simulink model "UZ_EnDat_be4_diffrework"  (R2023b)
settings: Solver=FixedStepDiscrete  StartTime=0  StopTime=0.002  RelTol=1e-3
model workspace (MAT data in the model file):
  Select = 0
libraries: hdlsllib x207, simulink x17, simulink_extras x3
(part 4 of 5)

== system UZ_EnDat_be4_diffrework/UZ_ENDAT/Subsystem/stalebootupfunction ==
  CLK : Inport
  RESET : Inport  Port=2
  CLKS2DATAFLOWCHG : Inport  Port=3
  CLK2ENDOFTRANSMISSION : Inport  Port=4
  VERYSLOWCLK : Inport  Port=5
  2CLKDELAY : Delay  DelayLength=0,  DelayLengthUpperLimit=1024
  2CLKDELAY2 : Delay  DelayLength=4  DelayLengthUpperLimit=1024
  Add : Sum  OutDataTypeStr=uint32  AccumDataTypeStr=uint32
  Add1 : Sum  OutDataTypeStr=uint32  AccumDataTypeStr=uint32
  BOOTOFFSETT2 : Constant  Value=19500  OutDataTypeStr=uint32  SampleTime=-1
  BOOTOFFSETT3 : Constant  Value=97501  OutDataTypeStr=uint32  SampleTime=-1
  CLKCNTERBOOTUP : Subsystem
      settings: LibrarySourceBlock=|
      | hdlsllib/Ports &
      | Subsystems/Subsystem
  Constant : Constant  Value=0xAAAA  OutDataTypeStr=uint16  SampleTime=-1
  Constant1 : Constant  OutDataTypeStr=boolean  SampleTime=-1
  Delay : Delay  DelayLength=1
  Logical Operator : Logic  Operator=NOT  AllPortsSameDT=off  OutDataTypeStr=boolean
  Logical Operator1 : Logic  AllPortsSameDT=off  OutDataTypeStr=boolean
  Logical Operator2 : Logic  Operator=OR  Inputs=3  AllPortsSameDT=off  OutDataTypeStr=boolean
  Logical Operator3 : Logic  AllPortsSameDT=off  OutDataTypeStr=boolean
  Logical Operator4 : Logic  Operator=OR  Inputs=3  AllPortsSameDT=off  OutDataTypeStr=boolean
  Logical Operator5 : Logic  Operator=OR  AllPortsSameDT=off  OutDataTypeStr=boolean
  ManualDeserializere : Subsystem
      settings: LibrarySourceBlock=|
      | hdlsllib/Ports &
      | Subsystems/Subsystem
  OUTPUTCONTROLCONTINIOUS : Subsystem
      settings: LibrarySourceBlock=|
      | hdlsllib/Ports &
      | Subsystems/Subsystem
  Relational Operator : RelationalOperator  Operator=<=  OutDataTypeStr=boolean  InputSameDT=off
  Relational Operator1 : RelationalOperator  Operator=<=  OutDataTypeStr=boolean  InputSameDT=off
  Relational Operator2 : RelationalOperator  Operator=>  OutDataTypeStr=boolean  InputSameDT=off
  TLOWOFFSET : Constant  Value=19501  OutDataTypeStr=uint32  SampleTime=-1
  Terminator : Terminator
  CLKOUT : Outport
  DATAOUT : Outport  Port=2
  BOOTUPCOMPLETE : Outport  Port=3  OutDataTypeStr=boolean
  DATAINV : Outport  Port=4
  wires:
  CLKS2DATAFLOWCHG/1 -> Add/1
  CLK2ENDOFTRANSMISSION/1 -> Add1/1
  OUTPUTCONTROLCONTINIOUS/1(CLKOFF) -> Delay/1, Logical Operator5/1
  Logical Operator/1 -> Logical Operator1/2, OUTPUTCONTROLCONTINIOUS/4(OPENCOM)
  OUTPUTCONTROLCONTINIOUS/3(RESETCNT) -> Terminator/1
  OUTPUTCONTROLCONTINIOUS/2(DATAINV) -> DATAINV/1
  CLK/1 -> CLKCNTERBOOTUP/1(CLK), ManualDeserializere/1(CLK)
  RESET/1 -> CLKCNTERBOOTUP/3(ResetCNT), Logical Operator5/2, Logical Operator4/1
  VERYSLOWCLK/1 -> ManualDeserializere/2(SLOWCLCK), CLKCNTERBOOTUP/2(CLK2CNT), Logical Operator1/1
  Logical Operator1/1 -> Logical Operator2/1
  Delay/1 -> Logical Operator/1
  Constant/1 -> ManualDeserializere/3(DATA)
  Constant1/1 -> ManualDeserializere/5(14)
  ManualDeserializere/1(valin) -> 2CLKDELAY/1
  CLKCNTERBOOTUP/1(CNT) -> Relational Operator2/1, Relational Operator1/1, Relational Operator/1, OUTPUTCONTROLCONTINIOUS/1(CLKCNT)
  Add1/1 -> OUTPUTCONTROLCONTINIOUS/3(CLK2ENDOFTRANSMISSION)
  Add/1 -> OUTPUTCONTROLCONTINIOUS/2(CLKS2DATAFLOWCHG)
  BOOTOFFSETT2/1 -> Relational Operator/2
  Relational Operator/1 -> Logical Operator4/3, Logical Operator2/2
  Logical Operator2/1 -> CLKOUT/1
  BOOTOFFSETT3/1 -> Add/2, Add1/2, Relational Operator1/2
  TLOWOFFSET/1 -> Relational Operator2/2
  Relational Operator1/1 -> Logical Operator3/2
  Relational Operator2/1 -> Logical Operator3/1
  Logical Operator3/1 -> Logical Operator2/3, Logical Operator4/2
  Logical Operator4/1 -> ManualDeserializere/4(reset)
  Logical Operator5/1 -> 2CLKDELAY2/1
  2CLKDELAY/1 -> DATAOUT/1
  2CLKDELAY2/1 -> BOOTUPCOMPLETE/1

== system UZ_EnDat_be4_diffrework/UZ_ENDAT/Subsystem2/ManualDeserializere ==
  CLK : Inport
  SLOWCLCK : Inport  Port=2
  DATA : Inport  Port=3
  reset : Inport  Port=4
  Constant3 : Constant  Value=0  OutDataTypeStr=boolean  SampleTime=-1
  Delay1 : Delay  DelayLength=1
  Multiport Switch : MultiPortSwitch  Inputs=6  DataPortForDefault=Additional data port  DiagnosticForDefault=None  SaturateOnIntegerOverflow=off  InputSameDT=off
  Terminator{1..10} (10 alike) : Terminator
  WORDTOBOOL : Subsystem  TreatAsAtomicUnit=on
  ramwatcher : Subsystem  TreatAsAtomicUnit=on
      settings: LibrarySourceBlock=|
      | hdlsllib/Ports &
      | Subsystems/Triggered
      | Subsystem
  valin : Outport
  wires:
  SLOWCLCK/1 -> ramwatcher/Trigger
  DATA/1 -> WORDTOBOOL/1(DATAIN)
  Multiport Switch/1 -> valin/1
  CLK/1 -> WORDTOBOOL/Trigger
  Delay1/1 -> ramwatcher/1(In1)
  Constant3/1 -> Multiport Switch/8
  reset/1 -> ramwatcher/2(reset)
  WORDTOBOOL/1(DATAOUT0) -> Multiport Switch/7
  WORDTOBOOL/2(DATAOUT1) -> Multiport Switch/6
  WORDTOBOOL/3(DATAOUT2) -> Multiport Switch/5
  WORDTOBOOL/4(DATAOUT3) -> Multiport Switch/4
  WORDTOBOOL/5(DATAOUT4) -> Multiport Switch/3
  WORDTOBOOL/6(DATAOUT5) -> Multiport Switch/2
  WORDTOBOOL/9(DATAOUT8) -> Terminator2/1
  WORDTOBOOL/10(DATAOUT9) -> Terminator3/1
  WORDTOBOOL/11(DATAOUT10) -> Terminator4/1
  WORDTOBOOL/12(DATAOUT11) -> Terminator5/1
  WORDTOBOOL/13(DATAOUT12) -> Terminator6/1
  WORDTOBOOL/14(DATAOUT13) -> Terminator7/1
  WORDTOBOOL/15(DATAOUT14) -> Terminator8/1
  WORDTOBOOL/16(DATAOUT15) -> Terminator9/1
  WORDTOBOOL/7(DATAOUT6) -> Terminator1/1
  WORDTOBOOL/8(DATAOUT7) -> Terminator10/1
  ramwatcher/1(SEL) -> Multiport Switch/1, Delay1/1

== system UZ_EnDat_be4_diffrework/UZ_ENDAT/responseslicer5/ENDAT23BITREVERSER ==
  in : Inport
  32BITREVERSE : Subsystem
  Bit Shift : hdlsllib/Logic and Bit Operations/Bit Shift  mode=Shift Right Logical  N=8
  Data Type Conversion : DataTypeConversion  OutDataTypeStr=uint32  RndMeth=Nearest  SaturateOnIntegerOverflow=off
  out : Outport
  wires:
  Bit Shift/1 -> out/1
  in/1 -> Data Type Conversion/1
  32BITREVERSE/1(out) -> Bit Shift/1
  Data Type Conversion/1 -> 32BITREVERSE/1(in)

== system UZ_EnDat_be4_diffrework/UZ_ENDAT/timingprovider/CLKCNTER_POSCNTR ==
  CLK : Inport
  CLK2CNT : Inport  Port=2
  ResetCNT : Inport  Port=3  OutDataTypeStr=boolean
  Delay1 : Delay  DelayLength=1
  Positional_Counter : Subsystem  TreatAsAtomicUnit=on
      settings: LibrarySourceBlock=|
      | hdlsllib/Ports &
      | Subsystems/Triggered
      | Subsystem
  SetZero32 : Subsystem  Commented=on
  SetZero32modified : Subsystem
  SetZero32modified1 : Subsystem
  CNT : Outport
  wires:
  CLK2CNT/1 -> Positional_Counter/Trigger
  Delay1/1 -> SetZero32modified1/1(valin), CNT/1
  SetZero32modified/1(valueout) -> Delay1/1
  CLK/1 -> SetZero32modified1/Trigger, SetZero32modified/Trigger
  Positional_Counter/1(divider) -> SetZero32modified/1(valin)
  ResetCNT/1 -> SetZero32modified1/2(setzero), SetZero32modified/2(setzero)
  SetZero32modified1/1(valueout) -> Positional_Counter/1(valueout)

== system UZ_EnDat_be4_diffrework/UZ_ENDAT/timingprovider/CLKCNTER_POSCNTR1 ==
  CLK : Inport
  CLK2CNT : Inport  Port=2
  ResetCNT : Inport  Port=3  OutDataTypeStr=boolean
  Delay1 : Delay  DelayLength=1
  Positional_Counter : Subsystem  TreatAsAtomicUnit=on
      settings: LibrarySourceBlock=|
      | hdlsllib/Ports &
      | Subsystems/Triggered
      | Subsystem
  SetZero32 : Subsystem  Commented=on
  SetZero32modified : Subsystem
  CNT : Outport
  wires:
  CLK2CNT/1 -> Positional_Counter/Trigger
  SetZero32modified/1(valueout) -> Delay1/1
  CLK/1 -> SetZero32modified/Trigger
  Positional_Counter/1(divider) -> SetZero32modified/1(valin)
  ResetCNT/1 -> SetZero32modified/2(setzero)
  Delay1/1 -> Positional_Counter/1(valueout), CNT/1

== system UZ_EnDat_be4_diffrework/UZ_ENDAT/timingprovider/Subsystem ==
  elapsed : Inport
  clkcnt : Inport  Port=2
  Compare To Constant1 : hdlsllib/Logic and Bit Operations/Compare To Constant  relop===  const=5  OutDataTypeStr=boolean
  Constant : Constant  Value=20  OutDataTypeStr=uint32  SampleTime=-1
  Delay1 : Delay  DelayLength=1
  Detect Increase : simulink/Logic and Bit Operations/Detect Increase  vinit=0.0  OutDataTypeStr=boolean
      settings: LibrarySourceBlock=|
      | hdlsllib/Logic and Bit
      | Operations/Detect
      | Increase
  Switch : Switch  Criteria=u2 > Threshold  SaturateOnIntegerOverflow=off  InputSameDT=off
  nsproduct : Product  OutDataTypeStr=uint32  RndMeth=Simplest  SaturateOnIntegerOverflow=on
  ns elapsed : Outport
  wires:
  Detect Increase/1 -> Switch/2
  clkcnt/1 -> Switch/1
  Switch/1 -> nsproduct/2, Delay1/1
  Delay1/1 -> Switch/3
  elapsed/1 -> Compare To Constant1/1
  nsproduct/1 -> ns elapsed/1  "ns elapsed"
  Constant/1 -> nsproduct/1
  Compare To Constant1/1 -> Detect Increase/1

== system UZ_EnDat_be4_diffrework/UZ_ENDAT/timingprovider/Subsystem1 ==
  elapsed : Inport
  clkcnt : Inport  Port=2
  Compare To Constant1 : hdlsllib/Logic and Bit Operations/Compare To Constant  relop===  const=4  OutDataTypeStr=boolean
  Constant : Constant  Value=20  OutDataTypeStr=uint32  SampleTime=-1
  Delay1 : Delay  DelayLength=1
  Detect Increase : simulink/Logic and Bit Operations/Detect Increase  vinit=0.0  OutDataTypeStr=boolean
      settings: LibrarySourceBlock=|
      | hdlsllib/Logic and Bit
      | Operations/Detect
      | Increase
  Switch : Switch  Criteria=u2 > Threshold  SaturateOnIntegerOverflow=off  InputSameDT=off
  nsproduct : Product  OutDataTypeStr=uint32  RndMeth=Simplest  SaturateOnIntegerOverflow=on
  ns elapsed : Outport
  wires:
  Detect Increase/1 -> Switch/2
  clkcnt/1 -> Switch/1
  Switch/1 -> nsproduct/2, Delay1/1
  Delay1/1 -> Switch/3
  elapsed/1 -> Compare To Constant1/1
  nsproduct/1 -> ns elapsed/1  "ns elapsed"
  Constant/1 -> nsproduct/1
  Compare To Constant1/1 -> Detect Increase/1

== system UZ_EnDat_be4_diffrework/UZ_ENDAT/timingprovider/Subsystem2 ==
  elapsed : Inport
  clkcnt : Inport  Port=2
  Compare To Constant1 : hdlsllib/Logic and Bit Operations/Compare To Constant  relop===  const=3  OutDataTypeStr=boolean
  Constant : Constant  Value=20  OutDataTypeStr=uint32  SampleTime=-1
  Delay1 : Delay  DelayLength=1
  Detect Increase : simulink/Logic and Bit Operations/Detect Increase  vinit=0.0  OutDataTypeStr=boolean
      settings: LibrarySourceBlock=|
      | hdlsllib/Logic and Bit
      | Operations/Detect
      | Increase
  Switch : Switch  Criteria=u2 > Threshold  SaturateOnIntegerOverflow=off  InputSameDT=off
  nsproduct : Product  OutDataTypeStr=uint32  RndMeth=Simplest  SaturateOnIntegerOverflow=on
  ns elapsed : Outport
  wires:
  Detect Increase/1 -> Switch/2
  clkcnt/1 -> Switch/1
  Switch/1 -> nsproduct/2, Delay1/1
  Delay1/1 -> Switch/3
  elapsed/1 -> Compare To Constant1/1
  nsproduct/1 -> ns elapsed/1  "ns elapsed"
  Constant/1 -> nsproduct/1
  Compare To Constant1/1 -> Detect Increase/1

== system UZ_EnDat_be4_diffrework/UZ_ENDAT/timingprovider/Subsystem3 ==
  elapsed : Inport
  clkcnt : Inport  Port=2
  Compare To Constant1 : hdlsllib/Logic and Bit Operations/Compare To Constant  relop===  const=2  OutDataTypeStr=boolean
  Constant : Constant  Value=20  OutDataTypeStr=uint32  SampleTime=-1
  Delay1 : Delay  DelayLength=1
  Detect Increase : simulink/Logic and Bit Operations/Detect Increase  vinit=0.0  OutDataTypeStr=boolean
      settings: LibrarySourceBlock=|
      | hdlsllib/Logic and Bit
      | Operations/Detect
      | Increase
  Switch : Switch  Criteria=u2 > Threshold  SaturateOnIntegerOverflow=off  InputSameDT=off
  nsproduct : Product  OutDataTypeStr=uint32  RndMeth=Simplest  SaturateOnIntegerOverflow=on
  ns elapsed : Outport
  wires:
  Detect Increase/1 -> Switch/2
  clkcnt/1 -> Switch/1
  Switch/1 -> nsproduct/2, Delay1/1
  Delay1/1 -> Switch/3
  elapsed/1 -> Compare To Constant1/1
  nsproduct/1 -> ns elapsed/1  "ns elapsed"
  Constant/1 -> nsproduct/1
  Compare To Constant1/1 -> Detect Increase/1

== system UZ_EnDat_be4_diffrework/UZ_ENDAT/timingprovider/Subsystem4 ==
  countclk : Inport
  reset : Inport  Port=2
  Delay : Delay  DelayLength=1
  Detect Increase : simulink/Logic and Bit Operations/Detect Increase  vinit=0.0  OutDataTypeStr=boolean
      settings: LibrarySourceBlock=|
      | hdlsllib/Logic and Bit
      | Operations/Detect
      | Increase
  HDL Counter : hdlsllib/Sources/HDL Counter  CountType=Count limited  CountInit=0  CountStep=1  CountMax=214748364  CountFromType=Initial value  CountFrom=0  CountResetPort=on  CountLoadPort=off  CountEnbPort=on  CountDirPort=off  CountHitOutputPort=off  CountDataType=Unsigned  CountWordLen=32  CountFracLen=0  CountSampTime=1
  Scope : Scope
  valin1 : Outport  InitialOutput=0
  wires:
  countclk/1 -> Detect Increase/1
  Detect Increase/1 -> HDL Counter/2
  reset/1 -> Delay/1
  HDL Counter/1 -> valin1/1, Scope/1
  Delay/1 -> HDL Counter/1

== system UZ_EnDat_be4_diffrework/UZ_ENDAT/CRC_Check/DFF1/JKFF ==
  SET : Inport
  CLK : Inport  Port=2
  J : Inport  Port=3
  RST : Inport  Port=4
  K : Inport  Port=5
  AND : Logic  Inputs=4  IconShape=distinctive  AllPortsSameDT=off  OutDataTypeStr=boolean
  AND1 : Logic  Inputs=4  IconShape=distinctive  AllPortsSameDT=off  OutDataTypeStr=boolean
  AND{2..5} (4 alike) : Logic  IconShape=distinctive  AllPortsSameDT=off  OutDataTypeStr=boolean
  Delay{,1..3} (4 alike) : Delay  DelayLength=1
  NOR : Logic  Operator=NOR  Inputs=4  IconShape=distinctive  AllPortsSameDT=off  OutDataTypeStr=boolean
  NOR1 : Logic  Operator=NOR  Inputs=4  IconShape=distinctive  AllPortsSameDT=off  OutDataTypeStr=boolean
  NOR2 : Logic  Operator=NOR  IconShape=distinctive  AllPortsSameDT=off  OutDataTypeStr=boolean
  NOR3 : Logic  Operator=NAND  IconShape=distinctive  AllPortsSameDT=off  OutDataTypeStr=boolean
  NOR4 : Logic  Operator=NOR  IconShape=distinctive  AllPortsSameDT=off  OutDataTypeStr=boolean
  NOR5 : Logic  Operator=NAND  IconShape=distinctive  AllPortsSameDT=off  OutDataTypeStr=boolean
  NOT : Logic  Operator=NOT  IconShape=distinctive  AllPortsSameDT=off  OutDataTypeStr=boolean
  NOT1 : Logic  Operator=NOT  IconShape=distinctive  AllPortsSameDT=off  OutDataTypeStr=boolean
  OR : Logic  Operator=OR  Inputs=3  IconShape=distinctive  AllPortsSameDT=off  OutDataTypeStr=boolean
  OQ : Outport
  NOQ : Outport  Port=2
  wires:
  RST/1 -> NOR4/2, NOR1/4
  J/1 -> OR/1, AND/2
  CLK/1 -> AND5/1, AND4/2, OR/2, NOT/1
  NOT/1 -> AND/3, AND1/2
  K/1 -> OR/3, AND1/3
  OR/1 -> AND1/1, NOT1/1, AND/4
  NOT1/1 -> AND2/1, AND3/2
  AND3/1 -> NOR/3
  AND/1 -> NOR/2
  AND2/1 -> NOR1/2
  AND1/1 -> NOR1/3
  SET/1 -> NOR2/1, NOR/1
  NOR/1 -> Delay/1
  NOR1/1 -> Delay1/1
  AND5/1 -> NOR2/2
  NOR2/1 -> NOR3/1
  AND4/1 -> NOR4/1
  NOR4/1 -> NOR5/2
  NOR3/1 -> Delay3/1
  NOR5/1 -> Delay2/1
  Delay/1 -> NOR1/1, AND4/1
  Delay1/1 -> NOR/4, AND5/2
  Delay2/1 -> NOR3/2, AND2/2, AND/1, NOQ/1
  Delay3/1 -> AND3/1, AND1/4, NOR5/1, OQ/1

== system UZ_EnDat_be4_diffrework/UZ_ENDAT/CRC_Check/DFF2/JKFF ==
  SET : Inport
  CLK : Inport  Port=2
  J : Inport  Port=3
  RST : Inport  Port=4
  K : Inport  Port=5
  AND : Logic  Inputs=4  IconShape=distinctive  AllPortsSameDT=off  OutDataTypeStr=boolean
  AND1 : Logic  Inputs=4  IconShape=distinctive  AllPortsSameDT=off  OutDataTypeStr=boolean
  AND{2..5} (4 alike) : Logic  IconShape=distinctive  AllPortsSameDT=off  OutDataTypeStr=boolean
  Delay{,1..3} (4 alike) : Delay  DelayLength=1
  NOR : Logic  Operator=NOR  Inputs=4  IconShape=distinctive  AllPortsSameDT=off  OutDataTypeStr=boolean
  NOR1 : Logic  Operator=NOR  Inputs=4  IconShape=distinctive  AllPortsSameDT=off  OutDataTypeStr=boolean
  NOR2 : Logic  Operator=NOR  IconShape=distinctive  AllPortsSameDT=off  OutDataTypeStr=boolean
  NOR3 : Logic  Operator=NAND  IconShape=distinctive  AllPortsSameDT=off  OutDataTypeStr=boolean
  NOR4 : Logic  Operator=NOR  IconShape=distinctive  AllPortsSameDT=off  OutDataTypeStr=boolean
  NOR5 : Logic  Operator=NAND  IconShape=distinctive  AllPortsSameDT=off  OutDataTypeStr=boolean
  NOT : Logic  Operator=NOT  IconShape=distinctive  AllPortsSameDT=off  OutDataTypeStr=boolean
  NOT1 : Logic  Operator=NOT  IconShape=distinctive  AllPortsSameDT=off  OutDataTypeStr=boolean
  OR : Logic  Operator=OR  Inputs=3  IconShape=distinctive  AllPortsSameDT=off  OutDataTypeStr=boolean
  OQ : Outport
  NOQ : Outport  Port=2
  wires:
  RST/1 -> NOR4/2, NOR1/4
  J/1 -> OR/1, AND/2
  CLK/1 -> AND5/1, AND4/2, OR/2, NOT/1
  NOT/1 -> AND/3, AND1/2
  K/1 -> OR/3, AND1/3
  OR/1 -> AND1/1, NOT1/1, AND/4
  NOT1/1 -> AND2/1, AND3/2
  AND3/1 -> NOR/3
  AND/1 -> NOR/2
  AND2/1 -> NOR1/2
  AND1/1 -> NOR1/3
  SET/1 -> NOR2/1, NOR/1
  NOR/1 -> Delay/1
  NOR1/1 -> Delay1/1
  AND5/1 -> NOR2/2
  NOR2/1 -> NOR3/1
  AND4/1 -> NOR4/1
  NOR4/1 -> NOR5/2
  NOR3/1 -> Delay3/1
  NOR5/1 -> Delay2/1
  Delay/1 -> NOR1/1, AND4/1
  Delay1/1 -> NOR/4, AND5/2
  Delay2/1 -> NOR3/2, AND2/2, AND/1, NOQ/1
  Delay3/1 -> AND3/1, AND1/4, NOR5/1, OQ/1

== system UZ_EnDat_be4_diffrework/UZ_ENDAT/CRC_Check/DFF3/JKFF ==
  SET : Inport
  CLK : Inport  Port=2
  J : Inport  Port=3
  RST : Inport  Port=4
  K : Inport  Port=5
  AND : Logic  Inputs=4  IconShape=distinctive  AllPortsSameDT=off  OutDataTypeStr=boolean
  AND1 : Logic  Inputs=4  IconShape=distinctive  AllPortsSameDT=off  OutDataTypeStr=boolean
  AND{2..5} (4 alike) : Logic  IconShape=distinctive  AllPortsSameDT=off  OutDataTypeStr=boolean
  Delay{,1..3} (4 alike) : Delay  DelayLength=1
  NOR : Logic  Operator=NOR  Inputs=4  IconShape=distinctive  AllPortsSameDT=off  OutDataTypeStr=boolean
  NOR1 : Logic  Operator=NOR  Inputs=4  IconShape=distinctive  AllPortsSameDT=off  OutDataTypeStr=boolean
  NOR2 : Logic  Operator=NOR  IconShape=distinctive  AllPortsSameDT=off  OutDataTypeStr=boolean
  NOR3 : Logic  Operator=NAND  IconShape=distinctive  AllPortsSameDT=off  OutDataTypeStr=boolean
  NOR4 : Logic  Operator=NOR  IconShape=distinctive  AllPortsSameDT=off  OutDataTypeStr=boolean
  NOR5 : Logic  Operator=NAND  IconShape=distinctive  AllPortsSameDT=off  OutDataTypeStr=boolean
  NOT : Logic  Operator=NOT  IconShape=distinctive  AllPortsSameDT=off  OutDataTypeStr=boolean
  NOT1 : Logic  Operator=NOT  IconShape=distinctive  AllPortsSameDT=off  OutDataTypeStr=boolean
  OR : Logic  Operator=OR  Inputs=3  IconShape=distinctive  AllPortsSameDT=off  OutDataTypeStr=boolean
  OQ : Outport
  NOQ : Outport  Port=2
  wires:
  RST/1 -> NOR4/2, NOR1/4
  J/1 -> OR/1, AND/2
  CLK/1 -> AND5/1, AND4/2, OR/2, NOT/1
  NOT/1 -> AND/3, AND1/2
  K/1 -> OR/3, AND1/3
  OR/1 -> AND1/1, NOT1/1, AND/4
  NOT1/1 -> AND2/1, AND3/2
  AND3/1 -> NOR/3
  AND/1 -> NOR/2
  AND2/1 -> NOR1/2
  AND1/1 -> NOR1/3
  SET/1 -> NOR2/1, NOR/1
  NOR/1 -> Delay/1
  NOR1/1 -> Delay1/1
  AND5/1 -> NOR2/2
  NOR2/1 -> NOR3/1
  AND4/1 -> NOR4/1
  NOR4/1 -> NOR5/2
  NOR3/1 -> Delay3/1
  NOR5/1 -> Delay2/1
  Delay/1 -> NOR1/1, AND4/1
  Delay1/1 -> NOR/4, AND5/2
  Delay2/1 -> NOR3/2, AND2/2, AND/1, NOQ/1
  Delay3/1 -> AND3/1, AND1/4, NOR5/1, OQ/1

== system UZ_EnDat_be4_diffrework/UZ_ENDAT/CRC_Check/DFF4/JKFF ==
  SET : Inport
  CLK : Inport  Port=2
  J : Inport  Port=3
  RST : Inport  Port=4
  K : Inport  Port=5
  AND : Logic  Inputs=4  IconShape=distinctive  AllPortsSameDT=off  OutDataTypeStr=boolean
  AND1 : Logic  Inputs=4  IconShape=distinctive  AllPortsSameDT=off  OutDataTypeStr=boolean
  AND{2..5} (4 alike) : Logic  IconShape=distinctive  AllPortsSameDT=off  OutDataTypeStr=boolean
  Delay{,1..3} (4 alike) : Delay  DelayLength=1
  NOR : Logic  Operator=NOR  Inputs=4  IconShape=distinctive  AllPortsSameDT=off  OutDataTypeStr=boolean
  NOR1 : Logic  Operator=NOR  Inputs=4  IconShape=distinctive  AllPortsSameDT=off  OutDataTypeStr=boolean
  NOR2 : Logic  Operator=NOR  IconShape=distinctive  AllPortsSameDT=off  OutDataTypeStr=boolean
  NOR3 : Logic  Operator=NAND  IconShape=distinctive  AllPortsSameDT=off  OutDataTypeStr=boolean
  NOR4 : Logic  Operator=NOR  IconShape=distinctive  AllPortsSameDT=off  OutDataTypeStr=boolean
  NOR5 : Logic  Operator=NAND  IconShape=distinctive  AllPortsSameDT=off  OutDataTypeStr=boolean
  NOT : Logic  Operator=NOT  IconShape=distinctive  AllPortsSameDT=off  OutDataTypeStr=boolean
  NOT1 : Logic  Operator=NOT  IconShape=distinctive  AllPortsSameDT=off  OutDataTypeStr=boolean
  OR : Logic  Operator=OR  Inputs=3  IconShape=distinctive  AllPortsSameDT=off  OutDataTypeStr=boolean
  OQ : Outport
  NOQ : Outport  Port=2
  wires:
  RST/1 -> NOR4/2, NOR1/4
  J/1 -> OR/1, AND/2
  CLK/1 -> AND5/1, AND4/2, OR/2, NOT/1
  NOT/1 -> AND/3, AND1/2
  K/1 -> OR/3, AND1/3
  OR/1 -> AND1/1, NOT1/1, AND/4
  NOT1/1 -> AND2/1, AND3/2
  AND3/1 -> NOR/3
  AND/1 -> NOR/2
  AND2/1 -> NOR1/2
  AND1/1 -> NOR1/3
  SET/1 -> NOR2/1, NOR/1
  NOR/1 -> Delay/1
  NOR1/1 -> Delay1/1
  AND5/1 -> NOR2/2
  NOR2/1 -> NOR3/1
  AND4/1 -> NOR4/1
  NOR4/1 -> NOR5/2
  NOR3/1 -> Delay3/1
  NOR5/1 -> Delay2/1
  Delay/1 -> NOR1/1, AND4/1
  Delay1/1 -> NOR/4, AND5/2
  Delay2/1 -> NOR3/2, AND2/2, AND/1, NOQ/1
  Delay3/1 -> AND3/1, AND1/4, NOR5/1, OQ/1

== system UZ_EnDat_be4_diffrework/UZ_ENDAT/CRC_Check/DFF5/JKFF ==
  SET : Inport
  CLK : Inport  Port=2
  J : Inport  Port=3
  RST : Inport  Port=4
  K : Inport  Port=5
  AND : Logic  Inputs=4  IconShape=distinctive  AllPortsSameDT=off  OutDataTypeStr=boolean
  AND1 : Logic  Inputs=4  IconShape=distinctive  AllPortsSameDT=off  OutDataTypeStr=boolean
  AND{2..5} (4 alike) : Logic  IconShape=distinctive  AllPortsSameDT=off  OutDataTypeStr=boolean
  Delay{,1..3} (4 alike) : Delay  DelayLength=1
  NOR : Logic  Operator=NOR  Inputs=4  IconShape=distinctive  AllPortsSameDT=off  OutDataTypeStr=boolean
  NOR1 : Logic  Operator=NOR  Inputs=4  IconShape=distinctive  AllPortsSameDT=off  OutDataTypeStr=boolean
  NOR2 : Logic  Operator=NOR  IconShape=distinctive  AllPortsSameDT=off  OutDataTypeStr=boolean
  NOR3 : Logic  Operator=NAND  IconShape=distinctive  AllPortsSameDT=off  OutDataTypeStr=boolean
  NOR4 : Logic  Operator=NOR  IconShape=distinctive  AllPortsSameDT=off  OutDataTypeStr=boolean
  NOR5 : Logic  Operator=NAND  IconShape=distinctive  AllPortsSameDT=off  OutDataTypeStr=boolean
  NOT : Logic  Operator=NOT  IconShape=distinctive  AllPortsSameDT=off  OutDataTypeStr=boolean
  NOT1 : Logic  Operator=NOT  IconShape=distinctive  AllPortsSameDT=off  OutDataTypeStr=boolean
  OR : Logic  Operator=OR  Inputs=3  IconShape=distinctive  AllPortsSameDT=off  OutDataTypeStr=boolean
  OQ : Outport
  NOQ : Outport  Port=2
  wires:
  RST/1 -> NOR4/2, NOR1/4
  J/1 -> OR/1, AND/2
  CLK/1 -> AND5/1, AND4/2, OR/2, NOT/1
  NOT/1 -> AND/3, AND1/2
  K/1 -> OR/3, AND1/3
  OR/1 -> AND1/1, NOT1/1, AND/4
  NOT1/1 -> AND2/1, AND3/2
  AND3/1 -> NOR/3
  AND/1 -> NOR/2
  AND2/1 -> NOR1/2
  AND1/1 -> NOR1/3
  SET/1 -> NOR2/1, NOR/1
  NOR/1 -> Delay/1
  NOR1/1 -> Delay1/1
  AND5/1 -> NOR2/2
  NOR2/1 -> NOR3/1
  AND4/1 -> NOR4/1
  NOR4/1 -> NOR5/2
  NOR3/1 -> Delay3/1
  NOR5/1 -> Delay2/1
  Delay/1 -> NOR1/1, AND4/1
  Delay1/1 -> NOR/4, AND5/2
  Delay2/1 -> NOR3/2, AND2/2, AND/1, NOQ/1
  Delay3/1 -> AND3/1, AND1/4, NOR5/1, OQ/1

== system UZ_EnDat_be4_diffrework/UZ_ENDAT/CRC_Check/DFF6/JKFF ==
  SET : Inport
  CLK : Inport  Port=2
  J : Inport  Port=3
  RST : Inport  Port=4
  K : Inport  Port=5
  AND : Logic  Inputs=4  IconShape=distinctive  AllPortsSameDT=off  OutDataTypeStr=boolean
  AND1 : Logic  Inputs=4  IconShape=distinctive  AllPortsSameDT=off  OutDataTypeStr=boolean
  AND{2..5} (4 alike) : Logic  IconShape=distinctive  AllPortsSameDT=off  OutDataTypeStr=boolean
  Delay{,1..3} (4 alike) : Delay  DelayLength=1
  NOR : Logic  Operator=NOR  Inputs=4  IconShape=distinctive  AllPortsSameDT=off  OutDataTypeStr=boolean
  NOR1 : Logic  Operator=NOR  Inputs=4  IconShape=distinctive  AllPortsSameDT=off  OutDataTypeStr=boolean
  NOR2 : Logic  Operator=NOR  IconShape=distinctive  AllPortsSameDT=off  OutDataTypeStr=boolean
  NOR3 : Logic  Operator=NAND  IconShape=distinctive  AllPortsSameDT=off  OutDataTypeStr=boolean
  NOR4 : Logic  Operator=NOR  IconShape=distinctive  AllPortsSameDT=off  OutDataTypeStr=boolean
  NOR5 : Logic  Operator=NAND  IconShape=distinctive  AllPortsSameDT=off  OutDataTypeStr=boolean
  NOT : Logic  Operator=NOT  IconShape=distinctive  AllPortsSameDT=off  OutDataTypeStr=boolean
  NOT1 : Logic  Operator=NOT  IconShape=distinctive  AllPortsSameDT=off  OutDataTypeStr=boolean
  OR : Logic  Operator=OR  Inputs=3  IconShape=distinctive  AllPortsSameDT=off  OutDataTypeStr=boolean
  OQ : Outport
  NOQ : Outport  Port=2
  wires:
  RST/1 -> NOR4/2, NOR1/4
  J/1 -> OR/1, AND/2
  CLK/1 -> AND5/1, AND4/2, OR/2, NOT/1
  NOT/1 -> AND/3, AND1/2
  K/1 -> OR/3, AND1/3
  OR/1 -> AND1/1, NOT1/1, AND/4
  NOT1/1 -> AND2/1, AND3/2
  AND3/1 -> NOR/3
  AND/1 -> NOR/2
  AND2/1 -> NOR1/2
  AND1/1 -> NOR1/3
  SET/1 -> NOR2/1, NOR/1
  NOR/1 -> Delay/1
  NOR1/1 -> Delay1/1
  AND5/1 -> NOR2/2
  NOR2/1 -> NOR3/1
  AND4/1 -> NOR4/1
  NOR4/1 -> NOR5/2
  NOR3/1 -> Delay3/1
  NOR5/1 -> Delay2/1
  Delay/1 -> NOR1/1, AND4/1
  Delay1/1 -> NOR/4, AND5/2
  Delay2/1 -> NOR3/2, AND2/2, AND/1, NOQ/1
  Delay3/1 -> AND3/1, AND1/4, NOR5/1, OQ/1

== system UZ_EnDat_be4_diffrework/UZ_ENDAT/INITIALOFF/CLKCNTER_FAST/Positional_Counter ==
  valueout : Inport  OutDataTypeStr=uint32
  Trigger : TriggerPort  TriggerType=either  VariantControl=(inherit)  InitialTriggerSignalState=zero
  Add : Sum  OutDataTypeStr=uint32  AccumDataTypeStr=uint32  InputSameDT=on  RndMeth=Simplest  SaturateOnIntegerOverflow=on
  Constant : Constant  OutDataTypeStr=uint32  SampleTime=-1
  divider : Outport  InitialOutput=0
  wires:
  valueout/1 -> Add/1
  Add/1 -> divider/1
  Constant/1 -> Add/2

== system UZ_EnDat_be4_diffrework/UZ_ENDAT/ManualSerialize/Storage1/prolonger ==
  in : Inport
  Delay4 : Delay  DelayLength=1
  Logical Operator5 : Logic  Operator=OR  AllPortsSameDT=off  OutDataTypeStr=boolean
  out : Outport
  wires:
  Logical Operator5/1 -> out/1
  in/1 -> Delay4/1, Logical Operator5/1
  Delay4/1 -> Logical Operator5/2

== system UZ_EnDat_be4_diffrework/UZ_ENDAT/ManualSerialize/Storage2/prolonger ==
  in : Inport
  Delay4 : Delay  DelayLength=1
  Logical Operator5 : Logic  Operator=OR  Inputs=3  AllPortsSameDT=off  OutDataTypeStr=boolean
  out : Outport
  wires:
  Logical Operator5/1 -> out/1
  in/1 -> Logical Operator5/3, Delay4/1, Logical Operator5/1
  Delay4/1 -> Logical Operator5/2

== system UZ_EnDat_be4_diffrework/UZ_ENDAT/ManualSerialize/nibblepadding6/padding ==
  in : Inport
  Bit Shift2 : hdlsllib/Logic and Bit Operations/Bit Shift  mode=Shift Right Logical  N=1
  Bit Slice2 : hdlsllib/Logic and Bit Operations/Bit Slice  lidx=0  ridx=0
  Data Type Conversion2 : DataTypeConversion  OutDataTypeStr=boolean  RndMeth=Nearest  SaturateOnIntegerOverflow=off
  Switch2 : Switch  Criteria=u2 > Threshold  SaturateOnIntegerOverflow=off  InputSameDT=off
  out : Outport
  wires:
  in/1 -> Bit Shift2/1, Switch2/1, Bit Slice2/1
  Bit Shift2/1 -> Switch2/3
  Data Type Conversion2/1 -> Switch2/2
  Bit Slice2/1 -> Data Type Conversion2/1
  Switch2/1 -> out/1

== system UZ_EnDat_be4_diffrework/UZ_ENDAT/ManualSerialize/nibblepadding6/padding1 ==
  in : Inport
  Bit Shift2 : hdlsllib/Logic and Bit Operations/Bit Shift  mode=Shift Right Logical  N=1
  Bit Slice2 : hdlsllib/Logic and Bit Operations/Bit Slice  lidx=0  ridx=0
  Data Type Conversion2 : DataTypeConversion  OutDataTypeStr=boolean  RndMeth=Nearest  SaturateOnIntegerOverflow=off
  Switch2 : Switch  Criteria=u2 > Threshold  SaturateOnIntegerOverflow=off  InputSameDT=off
  out : Outport
  wires:
  in/1 -> Bit Shift2/1, Switch2/1, Bit Slice2/1
  Bit Shift2/1 -> Switch2/3
  Data Type Conversion2/1 -> Switch2/2
  Bit Slice2/1 -> Data Type Conversion2/1
  Switch2/1 -> out/1

== system UZ_EnDat_be4_diffrework/UZ_ENDAT/ManualSerialize/nibblepadding6/padding2 ==
  in : Inport
  Bit Shift2 : hdlsllib/Logic and Bit Operations/Bit Shift  mode=Shift Right Logical  N=1
  Bit Slice2 : hdlsllib/Logic and Bit Operations/Bit Slice  lidx=0  ridx=0
  Data Type Conversion2 : DataTypeConversion  OutDataTypeStr=boolean  RndMeth=Nearest  SaturateOnIntegerOverflow=off
  Switch2 : Switch  Criteria=u2 > Threshold  SaturateOnIntegerOverflow=off  InputSameDT=off
  out : Outport
  wires:
  in/1 -> Bit Shift2/1, Switch2/1, Bit Slice2/1
  Bit Shift2/1 -> Switch2/3
  Data Type Conversion2/1 -> Switch2/2
  Bit Slice2/1 -> Data Type Conversion2/1
  Switch2/1 -> out/1

== system UZ_EnDat_be4_diffrework/UZ_ENDAT/ManualSerialize/nibblepadding6/padding3 ==
  in : Inport
  Bit Shift2 : hdlsllib/Logic and Bit Operations/Bit Shift  mode=Shift Right Logical  N=1
  Bit Slice2 : hdlsllib/Logic and Bit Operations/Bit Slice  lidx=0  ridx=0
  Data Type Conversion2 : DataTypeConversion  OutDataTypeStr=boolean  RndMeth=Nearest  SaturateOnIntegerOverflow=off
  Switch2 : Switch  Criteria=u2 > Threshold  SaturateOnIntegerOverflow=off  InputSameDT=off
  out : Outport
  wires:
  in/1 -> Bit Shift2/1, Switch2/1, Bit Slice2/1
  Bit Shift2/1 -> Switch2/3
  Data Type Conversion2/1 -> Switch2/2
  Bit Slice2/1 -> Data Type Conversion2/1
  Switch2/1 -> out/1

== system UZ_EnDat_be4_diffrework/UZ_ENDAT/RESPONSESLICER5X/19BITSLICER/responseslicer ==
  DATA : Inport  OutDataTypeStr=uint64
  Bit Slice1 : hdlsllib/Logic and Bit Operations/Bit Slice  lidx=2  ridx=2
  Bit Slice3 : hdlsllib/Logic and Bit Operations/Bit Slice  lidx=25  ridx=21
  Bit Slice4 : hdlsllib/Logic and Bit Operations/Bit Slice  lidx=20  ridx=2
  Data Type Conversion1 : DataTypeConversion  OutDataTypeStr=boolean  SaturateOnIntegerOverflow=off  RndMeth=Floor
  Data Type Conversion3 : DataTypeConversion  OutDataTypeStr=uint8  SaturateOnIntegerOverflow=off  RndMeth=Floor
  Data Type Conversion4 : DataTypeConversion  OutDataTypeStr=uint32  SaturateOnIntegerOverflow=off  RndMeth=Floor
  Terminator : Terminator
  CRC : Outport  OutDataTypeStr=uint8
  payload : Outport  Port=2  OutDataTypeStr=uint32
  error : Outport  Port=3  OutDataTypeStr=boolean
  wires:
  DATA/1 -> Terminator/1, Bit Slice1/1, Bit Slice4/1, Bit Slice3/1
  Bit Slice3/1 -> Data Type Conversion3/1
  Bit Slice4/1 -> Data Type Conversion4/1
  Data Type Conversion3/1 -> CRC/1
  Data Type Conversion4/1 -> payload/1
  Bit Slice1/1 -> Data Type Conversion1/1
  Data Type Conversion1/1 -> error/1

== system UZ_EnDat_be4_diffrework/UZ_ENDAT/RESPONSESLICER5X/19BITSLICER/responseslicer1 ==
  DATA : Inport  OutDataTypeStr=uint64
  Bit Slice1 : hdlsllib/Logic and Bit Operations/Bit Slice  lidx=2  ridx=2
  Bit Slice3 : hdlsllib/Logic and Bit Operations/Bit Slice  lidx=25  ridx=21
  Bit Slice4 : hdlsllib/Logic and Bit Operations/Bit Slice  lidx=20  ridx=2
  Data Type Conversion1 : DataTypeConversion  OutDataTypeStr=boolean  SaturateOnIntegerOverflow=off  RndMeth=Floor
  Data Type Conversion3 : DataTypeConversion  OutDataTypeStr=uint8  SaturateOnIntegerOverflow=off  RndMeth=Floor
  Data Type Conversion4 : DataTypeConversion  OutDataTypeStr=uint32  SaturateOnIntegerOverflow=off  RndMeth=Floor
  Terminator : Terminator
  CRC : Outport  OutDataTypeStr=uint8
  payload : Outport  Port=2  OutDataTypeStr=uint32
  error : Outport  Port=3  OutDataTypeStr=boolean
  wires:
  DATA/1 -> Terminator/1, Bit Slice1/1, Bit Slice4/1, Bit Slice3/1
  Bit Slice3/1 -> Data Type Conversion3/1
  Bit Slice4/1 -> Data Type Conversion4/1
  Data Type Conversion3/1 -> CRC/1
  Data Type Conversion4/1 -> payload/1
  Bit Slice1/1 -> Data Type Conversion1/1
  Data Type Conversion1/1 -> error/1

== system UZ_EnDat_be4_diffrework/UZ_ENDAT/RESPONSESLICER5X/19BITSLICER/responseslicer2 ==
  DATA : Inport  OutDataTypeStr=uint64
  Bit Slice1 : hdlsllib/Logic and Bit Operations/Bit Slice  lidx=2  ridx=2
  Bit Slice3 : hdlsllib/Logic and Bit Operations/Bit Slice  lidx=25  ridx=21
  Bit Slice4 : hdlsllib/Logic and Bit Operations/Bit Slice  lidx=20  ridx=2
  Data Type Conversion1 : DataTypeConversion  OutDataTypeStr=boolean  SaturateOnIntegerOverflow=off  RndMeth=Floor
  Data Type Conversion3 : DataTypeConversion  OutDataTypeStr=uint8  SaturateOnIntegerOverflow=off  RndMeth=Floor
  Data Type Conversion4 : DataTypeConversion  OutDataTypeStr=uint32  SaturateOnIntegerOverflow=off  RndMeth=Floor
  Terminator : Terminator
  CRC : Outport  OutDataTypeStr=uint8
  payload : Outport  Port=2  OutDataTypeStr=uint32
  error : Outport  Port=3  OutDataTypeStr=boolean
  wires:
  DATA/1 -> Terminator/1, Bit Slice1/1, Bit Slice4/1, Bit Slice3/1
  Bit Slice3/1 -> Data Type Conversion3/1
  Bit Slice4/1 -> Data Type Conversion4/1
  Data Type Conversion3/1 -> CRC/1
  Data Type Conversion4/1 -> payload/1
  Bit Slice1/1 -> Data Type Conversion1/1
  Data Type Conversion1/1 -> error/1

== system UZ_EnDat_be4_diffrework/UZ_ENDAT/RESPONSESLICER5X/19BITSLICER/responseslicer3 ==
  DATA : Inport  OutDataTypeStr=uint64
  Bit Slice1 : hdlsllib/Logic and Bit Operations/Bit Slice  lidx=2  ridx=2
  Bit Slice3 : hdlsllib/Logic and Bit Operations/Bit Slice  lidx=25  ridx=21
  Bit Slice4 : hdlsllib/Logic and Bit Operations/Bit Slice  lidx=20  ridx=2
  Data Type Conversion1 : DataTypeConversion  OutDataTypeStr=boolean  SaturateOnIntegerOverflow=off  RndMeth=Floor
  Data Type Conversion3 : DataTypeConversion  OutDataTypeStr=uint8  SaturateOnIntegerOverflow=off  RndMeth=Floor
  Data Type Conversion4 : DataTypeConversion  OutDataTypeStr=uint32  SaturateOnIntegerOverflow=off  RndMeth=Floor
  Terminator : Terminator
  CRC : Outport  OutDataTypeStr=uint8
  payload : Outport  Port=2  OutDataTypeStr=uint32
  error : Outport  Port=3  OutDataTypeStr=boolean
  wires:
  DATA/1 -> Terminator/1, Bit Slice1/1, Bit Slice4/1, Bit Slice3/1
  Bit Slice3/1 -> Data Type Conversion3/1
  Bit Slice4/1 -> Data Type Conversion4/1
  Data Type Conversion3/1 -> CRC/1
  Data Type Conversion4/1 -> payload/1
  Bit Slice1/1 -> Data Type Conversion1/1
  Data Type Conversion1/1 -> error/1

== system UZ_EnDat_be4_diffrework/UZ_ENDAT/RESPONSESLICER5X/19BITSLICER/responseslicer4 ==
  DATA : Inport  OutDataTypeStr=uint64
  Bit Slice1 : hdlsllib/Logic and Bit Operations/Bit Slice  lidx=2  ridx=2
  Bit Slice3 : hdlsllib/Logic and Bit Operations/Bit Slice  lidx=25  ridx=21
  Bit Slice4 : hdlsllib/Logic and Bit Operations/Bit Slice  lidx=20  ridx=2
  Data Type Conversion1 : DataTypeConversion  OutDataTypeStr=boolean  SaturateOnIntegerOverflow=off  RndMeth=Floor
  Data Type Conversion3 : DataTypeConversion  OutDataTypeStr=uint8  SaturateOnIntegerOverflow=off  RndMeth=Floor
  Data Type Conversion4 : DataTypeConversion  OutDataTypeStr=uint32  SaturateOnIntegerOverflow=off  RndMeth=Floor
  Terminator : Terminator
  CRC : Outport  OutDataTypeStr=uint8
  payload : Outport  Port=2  OutDataTypeStr=uint32
  error : Outport  Port=3  OutDataTypeStr=boolean
  wires:
  DATA/1 -> Terminator/1, Bit Slice1/1, Bit Slice4/1, Bit Slice3/1
  Bit Slice3/1 -> Data Type Conversion3/1
  Bit Slice4/1 -> Data Type Conversion4/1
  Data Type Conversion3/1 -> CRC/1
  Data Type Conversion4/1 -> payload/1
  Bit Slice1/1 -> Data Type Conversion1/1
  Data Type Conversion1/1 -> error/1

== system UZ_EnDat_be4_diffrework/UZ_ENDAT/RESPONSESLICER5X/21BITSLICER/responseslicer ==
  DATA : Inport  OutDataTypeStr=uint64
  Bit Slice1 : hdlsllib/Logic and Bit Operations/Bit Slice  lidx=2  ridx=2
  Bit Slice3 : hdlsllib/Logic and Bit Operations/Bit Slice  lidx=27  ridx=23
  Bit Slice4 : hdlsllib/Logic and Bit Operations/Bit Slice  lidx=22  ridx=2
  Data Type Conversion1 : DataTypeConversion  OutDataTypeStr=boolean  SaturateOnIntegerOverflow=off  RndMeth=Floor
  Data Type Conversion3 : DataTypeConversion  OutDataTypeStr=uint8  SaturateOnIntegerOverflow=off  RndMeth=Floor
  Data Type Conversion4 : DataTypeConversion  OutDataTypeStr=uint32  SaturateOnIntegerOverflow=off  RndMeth=Floor
  Terminator : Terminator
  CRC : Outport  OutDataTypeStr=uint8
  payload : Outport  Port=2  OutDataTypeStr=uint32
  error : Outport  Port=3  OutDataTypeStr=boolean
  wires:
  DATA/1 -> Terminator/1, Bit Slice1/1, Bit Slice4/1, Bit Slice3/1
  Bit Slice3/1 -> Data Type Conversion3/1
  Bit Slice4/1 -> Data Type Conversion4/1
  Data Type Conversion3/1 -> CRC/1
  Data Type Conversion4/1 -> payload/1
  Bit Slice1/1 -> Data Type Conversion1/1
  Data Type Conversion1/1 -> error/1

== system UZ_EnDat_be4_diffrework/UZ_ENDAT/RESPONSESLICER5X/21BITSLICER/responseslicer1 ==
  DATA : Inport  OutDataTypeStr=uint64
  Bit Slice1 : hdlsllib/Logic and Bit Operations/Bit Slice  lidx=2  ridx=2
  Bit Slice3 : hdlsllib/Logic and Bit Operations/Bit Slice  lidx=27  ridx=23
  Bit Slice4 : hdlsllib/Logic and Bit Operations/Bit Slice  lidx=22  ridx=2
  Data Type Conversion1 : DataTypeConversion  OutDataTypeStr=boolean  SaturateOnIntegerOverflow=off  RndMeth=Floor
  Data Type Conversion3 : DataTypeConversion  OutDataTypeStr=uint8  SaturateOnIntegerOverflow=off  RndMeth=Floor
  Data Type Conversion4 : DataTypeConversion  OutDataTypeStr=uint32  SaturateOnIntegerOverflow=off  RndMeth=Floor
  Terminator : Terminator
  CRC : Outport  OutDataTypeStr=uint8
  payload : Outport  Port=2  OutDataTypeStr=uint32
  error : Outport  Port=3  OutDataTypeStr=boolean
  wires:
  DATA/1 -> Terminator/1, Bit Slice1/1, Bit Slice4/1, Bit Slice3/1
  Bit Slice3/1 -> Data Type Conversion3/1
  Bit Slice4/1 -> Data Type Conversion4/1
  Data Type Conversion3/1 -> CRC/1
  Data Type Conversion4/1 -> payload/1
  Bit Slice1/1 -> Data Type Conversion1/1
  Data Type Conversion1/1 -> error/1

== system UZ_EnDat_be4_diffrework/UZ_ENDAT/RESPONSESLICER5X/21BITSLICER/responseslicer2 ==
  DATA : Inport  OutDataTypeStr=uint64
  Bit Slice1 : hdlsllib/Logic and Bit Operations/Bit Slice  lidx=2  ridx=2
  Bit Slice3 : hdlsllib/Logic and Bit Operations/Bit Slice  lidx=27  ridx=23
  Bit Slice4 : hdlsllib/Logic and Bit Operations/Bit Slice  lidx=22  ridx=2
  Data Type Conversion1 : DataTypeConversion  OutDataTypeStr=boolean  SaturateOnIntegerOverflow=off  RndMeth=Floor
  Data Type Conversion3 : DataTypeConversion  OutDataTypeStr=uint8  SaturateOnIntegerOverflow=off  RndMeth=Floor
  Data Type Conversion4 : DataTypeConversion  OutDataTypeStr=uint32  SaturateOnIntegerOverflow=off  RndMeth=Floor
  Terminator : Terminator
  CRC : Outport  OutDataTypeStr=uint8
  payload : Outport  Port=2  OutDataTypeStr=uint32
  error : Outport  Port=3  OutDataTypeStr=boolean
  wires:
  DATA/1 -> Terminator/1, Bit Slice1/1, Bit Slice4/1, Bit Slice3/1
  Bit Slice3/1 -> Data Type Conversion3/1
  Bit Slice4/1 -> Data Type Conversion4/1
  Data Type Conversion3/1 -> CRC/1
  Data Type Conversion4/1 -> payload/1
  Bit Slice1/1 -> Data Type Conversion1/1
  Data Type Conversion1/1 -> error/1

== system UZ_EnDat_be4_diffrework/UZ_ENDAT/RESPONSESLICER5X/21BITSLICER/responseslicer3 ==
  DATA : Inport  OutDataTypeStr=uint64
  Bit Slice1 : hdlsllib/Logic and Bit Operations/Bit Slice  lidx=2  ridx=2
  Bit Slice3 : hdlsllib/Logic and Bit Operations/Bit Slice  lidx=27  ridx=23
  Bit Slice4 : hdlsllib/Logic and Bit Operations/Bit Slice  lidx=22  ridx=2
  Data Type Conversion1 : DataTypeConversion  OutDataTypeStr=boolean  SaturateOnIntegerOverflow=off  RndMeth=Floor
  Data Type Conversion3 : DataTypeConversion  OutDataTypeStr=uint8  SaturateOnIntegerOverflow=off  RndMeth=Floor
  Data Type Conversion4 : DataTypeConversion  OutDataTypeStr=uint32  SaturateOnIntegerOverflow=off  RndMeth=Floor
  Terminator : Terminator
  CRC : Outport  OutDataTypeStr=uint8
  payload : Outport  Port=2  OutDataTypeStr=uint32
  error : Outport  Port=3  OutDataTypeStr=boolean
  wires:
  DATA/1 -> Terminator/1, Bit Slice1/1, Bit Slice4/1, Bit Slice3/1
  Bit Slice3/1 -> Data Type Conversion3/1
  Bit Slice4/1 -> Data Type Conversion4/1
  Data Type Conversion3/1 -> CRC/1
  Data Type Conversion4/1 -> payload/1
  Bit Slice1/1 -> Data Type Conversion1/1
  Data Type Conversion1/1 -> error/1

== system UZ_EnDat_be4_diffrework/UZ_ENDAT/RESPONSESLICER5X/21BITSLICER/responseslicer4 ==
  DATA : Inport  OutDataTypeStr=uint64
  Bit Slice1 : hdlsllib/Logic and Bit Operations/Bit Slice  lidx=2  ridx=2
  Bit Slice3 : hdlsllib/Logic and Bit Operations/Bit Slice  lidx=27  ridx=23
  Bit Slice4 : hdlsllib/Logic and Bit Operations/Bit Slice  lidx=22  ridx=2
  Data Type Conversion1 : DataTypeConversion  OutDataTypeStr=boolean  SaturateOnIntegerOverflow=off  RndMeth=Floor
  Data Type Conversion3 : DataTypeConversion  OutDataTypeStr=uint8  SaturateOnIntegerOverflow=off  RndMeth=Floor
  Data Type Conversion4 : DataTypeConversion  OutDataTypeStr=uint32  SaturateOnIntegerOverflow=off  RndMeth=Floor
  Terminator : Terminator
  CRC : Outport  OutDataTypeStr=uint8
  payload : Outport  Port=2  OutDataTypeStr=uint32
  error : Outport  Port=3  OutDataTypeStr=boolean
  wires:
  DATA/1 -> Terminator/1, Bit Slice1/1, Bit Slice4/1, Bit Slice3/1
  Bit Slice3/1 -> Data Type Conversion3/1
  Bit Slice4/1 -> Data Type Conversion4/1
  Data Type Conversion3/1 -> CRC/1
  Data Type Conversion4/1 -> payload/1
  Bit Slice1/1 -> Data Type Conversion1/1
  Data Type Conversion1/1 -> error/1

== system UZ_EnDat_be4_diffrework/UZ_ENDAT/RESPONSESLICER5X/23BITSLICER/responseslicer ==
  DATA : Inport  OutDataTypeStr=uint64
  Bit Slice1 : hdlsllib/Logic and Bit Operations/Bit Slice  lidx=2  ridx=2
  Bit Slice3 : hdlsllib/Logic and Bit Operations/Bit Slice  lidx=29  ridx=25
  Bit Slice4 : hdlsllib/Logic and Bit Operations/Bit Slice  lidx=24  ridx=2
  Data Type Conversion1 : DataTypeConversion  OutDataTypeStr=boolean  SaturateOnIntegerOverflow=off  RndMeth=Floor
  Data Type Conversion3 : DataTypeConversion  OutDataTypeStr=uint8  SaturateOnIntegerOverflow=off  RndMeth=Floor
  Data Type Conversion4 : DataTypeConversion  OutDataTypeStr=uint32  SaturateOnIntegerOverflow=off  RndMeth=Floor
  Terminator : Terminator
  CRC : Outport  OutDataTypeStr=uint8
  payload : Outport  Port=2  OutDataTypeStr=uint32
  error : Outport  Port=3  OutDataTypeStr=boolean
  wires:
  DATA/1 -> Terminator/1, Bit Slice1/1, Bit Slice4/1, Bit Slice3/1
  Bit Slice3/1 -> Data Type Conversion3/1
  Bit Slice4/1 -> Data Type Conversion4/1
  Data Type Conversion3/1 -> CRC/1
  Data Type Conversion4/1 -> payload/1
  Bit Slice1/1 -> Data Type Conversion1/1
  Data Type Conversion1/1 -> error/1

== system UZ_EnDat_be4_diffrework/UZ_ENDAT/RESPONSESLICER5X/23BITSLICER/responseslicer1 ==
  DATA : Inport  OutDataTypeStr=uint64
  Bit Slice1 : hdlsllib/Logic and Bit Operations/Bit Slice  lidx=2  ridx=2
  Bit Slice3 : hdlsllib/Logic and Bit Operations/Bit Slice  lidx=29  ridx=25
  Bit Slice4 : hdlsllib/Logic and Bit Operations/Bit Slice  lidx=24  ridx=2
  Data Type Conversion1 : DataTypeConversion  OutDataTypeStr=boolean  SaturateOnIntegerOverflow=off  RndMeth=Floor
  Data Type Conversion3 : DataTypeConversion  OutDataTypeStr=uint8  SaturateOnIntegerOverflow=off  RndMeth=Floor
  Data Type Conversion4 : DataTypeConversion  OutDataTypeStr=uint32  SaturateOnIntegerOverflow=off  RndMeth=Floor
  Terminator : Terminator
  CRC : Outport  OutDataTypeStr=uint8
  payload : Outport  Port=2  OutDataTypeStr=uint32
  error : Outport  Port=3  OutDataTypeStr=boolean
  wires:
  DATA/1 -> Terminator/1, Bit Slice1/1, Bit Slice4/1, Bit Slice3/1
  Bit Slice3/1 -> Data Type Conversion3/1
  Bit Slice4/1 -> Data Type Conversion4/1
  Data Type Conversion3/1 -> CRC/1
  Data Type Conversion4/1 -> payload/1
  Bit Slice1/1 -> Data Type Conversion1/1
  Data Type Conversion1/1 -> error/1

== system UZ_EnDat_be4_diffrework/UZ_ENDAT/RESPONSESLICER5X/23BITSLICER/responseslicer2 ==
  DATA : Inport  OutDataTypeStr=uint64
  Bit Slice1 : hdlsllib/Logic and Bit Operations/Bit Slice  lidx=2  ridx=2
  Bit Slice3 : hdlsllib/Logic and Bit Operations/Bit Slice  lidx=29  ridx=25
  Bit Slice4 : hdlsllib/Logic and Bit Operations/Bit Slice  lidx=24  ridx=2
  Data Type Conversion1 : DataTypeConversion  OutDataTypeStr=boolean  SaturateOnIntegerOverflow=off  RndMeth=Floor
  Data Type Conversion3 : DataTypeConversion  OutDataTypeStr=uint8  SaturateOnIntegerOverflow=off  RndMeth=Floor
  Data Type Conversion4 : DataTypeConversion  OutDataTypeStr=uint32  SaturateOnIntegerOverflow=off  RndMeth=Floor
  Terminator : Terminator
  CRC : Outport  OutDataTypeStr=uint8
  payload : Outport  Port=2  OutDataTypeStr=uint32
  error : Outport  Port=3  OutDataTypeStr=boolean
  wires:
  DATA/1 -> Terminator/1, Bit Slice1/1, Bit Slice4/1, Bit Slice3/1
  Bit Slice3/1 -> Data Type Conversion3/1
  Bit Slice4/1 -> Data Type Conversion4/1
  Data Type Conversion3/1 -> CRC/1
  Data Type Conversion4/1 -> payload/1
  Bit Slice1/1 -> Data Type Conversion1/1
  Data Type Conversion1/1 -> error/1

== system UZ_EnDat_be4_diffrework/UZ_ENDAT/RESPONSESLICER5X/23BITSLICER/responseslicer3 ==
  DATA : Inport  OutDataTypeStr=uint64
  Bit Slice1 : hdlsllib/Logic and Bit Operations/Bit Slice  lidx=2  ridx=2
  Bit Slice3 : hdlsllib/Logic and Bit Operations/Bit Slice  lidx=29  ridx=25
  Bit Slice4 : hdlsllib/Logic and Bit Operations/Bit Slice  lidx=24  ridx=2
  Data Type Conversion1 : DataTypeConversion  OutDataTypeStr=boolean  SaturateOnIntegerOverflow=off  RndMeth=Floor
  Data Type Conversion3 : DataTypeConversion  OutDataTypeStr=uint8  SaturateOnIntegerOverflow=off  RndMeth=Floor
  Data Type Conversion4 : DataTypeConversion  OutDataTypeStr=uint32  SaturateOnIntegerOverflow=off  RndMeth=Floor
  Terminator : Terminator
  CRC : Outport  OutDataTypeStr=uint8
  payload : Outport  Port=2  OutDataTypeStr=uint32
  error : Outport  Port=3  OutDataTypeStr=boolean
  wires:
  DATA/1 -> Terminator/1, Bit Slice1/1, Bit Slice4/1, Bit Slice3/1
  Bit Slice3/1 -> Data Type Conversion3/1
  Bit Slice4/1 -> Data Type Conversion4/1
  Data Type Conversion3/1 -> CRC/1
  Data Type Conversion4/1 -> payload/1
  Bit Slice1/1 -> Data Type Conversion1/1
  Data Type Conversion1/1 -> error/1

== system UZ_EnDat_be4_diffrework/UZ_ENDAT/RESPONSESLICER5X/23BITSLICER/responseslicer4 ==
  DATA : Inport  OutDataTypeStr=uint64
  Bit Slice1 : hdlsllib/Logic and Bit Operations/Bit Slice  lidx=2  ridx=2
  Bit Slice3 : hdlsllib/Logic and Bit Operations/Bit Slice  lidx=29  ridx=25
  Bit Slice4 : hdlsllib/Logic and Bit Operations/Bit Slice  lidx=24  ridx=2
  Data Type Conversion1 : DataTypeConversion  OutDataTypeStr=boolean  SaturateOnIntegerOverflow=off  RndMeth=Floor
  Data Type Conversion3 : DataTypeConversion  OutDataTypeStr=uint8  SaturateOnIntegerOverflow=off  RndMeth=Floor
  Data Type Conversion4 : DataTypeConversion  OutDataTypeStr=uint32  SaturateOnIntegerOverflow=off  RndMeth=Floor
  Terminator : Terminator
  CRC : Outport  OutDataTypeStr=uint8
  payload : Outport  Port=2  OutDataTypeStr=uint32
  error : Outport  Port=3  OutDataTypeStr=boolean
  wires:
  DATA/1 -> Terminator/1, Bit Slice1/1, Bit Slice4/1, Bit Slice3/1
  Bit Slice3/1 -> Data Type Conversion3/1
  Bit Slice4/1 -> Data Type Conversion4/1
  Data Type Conversion3/1 -> CRC/1
  Data Type Conversion4/1 -> payload/1
  Bit Slice1/1 -> Data Type Conversion1/1
  Data Type Conversion1/1 -> error/1

== system UZ_EnDat_be4_diffrework/UZ_ENDAT/RESPONSESLICER5X/25BITSLICER/responseslicer ==
  DATA : Inport  OutDataTypeStr=uint64
  Bit Slice1 : hdlsllib/Logic and Bit Operations/Bit Slice  lidx=2  ridx=2
  Bit Slice3 : hdlsllib/Logic and Bit Operations/Bit Slice  lidx=31  ridx=27
  Bit Slice4 : hdlsllib/Logic and Bit Operations/Bit Slice  lidx=26  ridx=2
  Data Type Conversion1 : DataTypeConversion  OutDataTypeStr=boolean  SaturateOnIntegerOverflow=off  RndMeth=Floor
  Data Type Conversion3 : DataTypeConversion  OutDataTypeStr=uint8  SaturateOnIntegerOverflow=off  RndMeth=Floor
  Data Type Conversion4 : DataTypeConversion  OutDataTypeStr=uint32  SaturateOnIntegerOverflow=off  RndMeth=Floor
  Terminator : Terminator
  CRC : Outport  OutDataTypeStr=uint8
  payload : Outport  Port=2  OutDataTypeStr=uint32
  error : Outport  Port=3  OutDataTypeStr=boolean
  wires:
  DATA/1 -> Terminator/1, Bit Slice1/1, Bit Slice4/1, Bit Slice3/1
  Bit Slice3/1 -> Data Type Conversion3/1
  Bit Slice4/1 -> Data Type Conversion4/1
  Data Type Conversion3/1 -> CRC/1
  Data Type Conversion4/1 -> payload/1
  Bit Slice1/1 -> Data Type Conversion1/1
  Data Type Conversion1/1 -> error/1

== system UZ_EnDat_be4_diffrework/UZ_ENDAT/RESPONSESLICER5X/25BITSLICER/responseslicer1 ==
  DATA : Inport  OutDataTypeStr=uint64
  Bit Slice1 : hdlsllib/Logic and Bit Operations/Bit Slice  lidx=2  ridx=2
  Bit Slice3 : hdlsllib/Logic and Bit Operations/Bit Slice  lidx=31  ridx=27
  Bit Slice4 : hdlsllib/Logic and Bit Operations/Bit Slice  lidx=26  ridx=2
  Data Type Conversion1 : DataTypeConversion  OutDataTypeStr=boolean  SaturateOnIntegerOverflow=off  RndMeth=Floor
  Data Type Conversion3 : DataTypeConversion  OutDataTypeStr=uint8  SaturateOnIntegerOverflow=off  RndMeth=Floor
  Data Type Conversion4 : DataTypeConversion  OutDataTypeStr=uint32  SaturateOnIntegerOverflow=off  RndMeth=Floor
  Terminator : Terminator
  CRC : Outport  OutDataTypeStr=uint8
  payload : Outport  Port=2  OutDataTypeStr=uint32
  error : Outport  Port=3  OutDataTypeStr=boolean
  wires:
  DATA/1 -> Terminator/1, Bit Slice1/1, Bit Slice4/1, Bit Slice3/1
  Bit Slice3/1 -> Data Type Conversion3/1
  Bit Slice4/1 -> Data Type Conversion4/1
  Data Type Conversion3/1 -> CRC/1
  Data Type Conversion4/1 -> payload/1
  Bit Slice1/1 -> Data Type Conversion1/1
  Data Type Conversion1/1 -> error/1
